simulink model "plant"  (R2023a)
settings: Solver=FixedStepAuto  StartTime=0.0  StopTime=10.0  FixedStep=0.01  RelTol=1e-3
libraries: shared6dof x1, simulink x1
settings Model: Creator=timme  LastModifiedBy=timme
settings OptimizationCC: BlockReduction=off  DefaultParameterBehavior=Inlined  BufferReuse=off

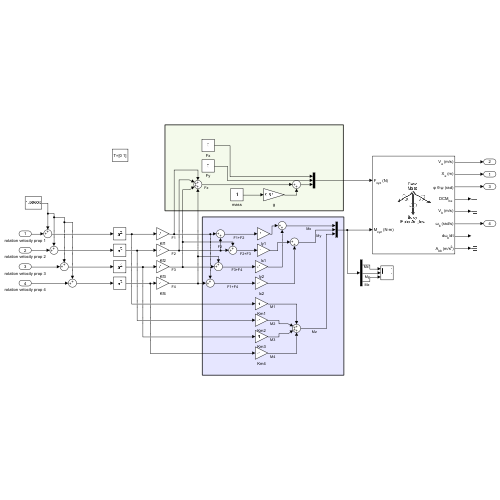
[thumbnail: Simulink's stored preview of the top-level diagram]
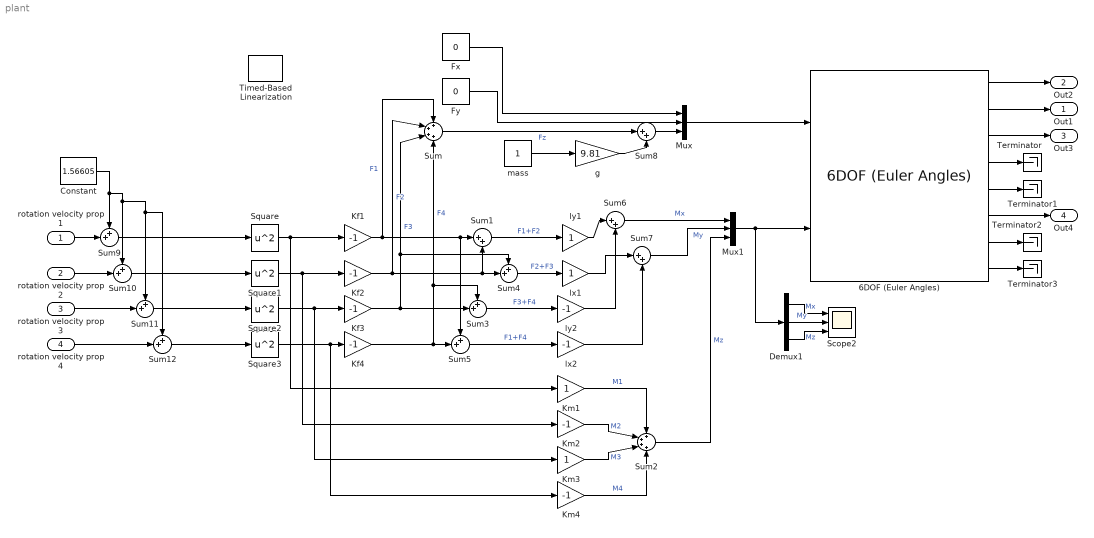
== system plant ==
  rotation velocity prop 1 : Inport
  rotation velocity prop 2 : Inport  Port=2
  rotation velocity prop 3 : Inport  Port=3
  rotation velocity prop 4 : Inport  Port=4
  6DOF (Euler Angles) : shared6dof/6DOF (Euler Angles)  units=Metric (MKS)  mtype=Fixed  rep=Euler Angles  xme_0=[0 0 0]  Vm_0=[0 0 0]  eul_0=[0 0 0]  pm_0=[0 0 0]  mass_0=1.0  mass_e=0.5  mass_f=2.0  inertia=eye(3)  inertia_e=eye(3)  inertia_f=2*eye(3)  k_quat=1.0  vre_flag=on  abi_flag=off  aMode=0  xme_statename=''  Vm_statename=''  eul_statename=''  quat_statename=''  pm_statename=''  mass_statename=''
  Constant : Constant  Value=1.56605
  Demux1 : Demux  Outputs=3
  Fx : Constant  Value=0
  Fy : Constant  Value=0
  Kf{1..4} (4 alike) : Gain  Gain=-1
  Km1 : Gain
  Km2 : Gain  Gain=-1
  Km3 : Gain
  Km4 : Gain  Gain=-1
  Mux : Mux  Inputs=3
  Mux1 : Mux  Inputs=3
  Scope2 : Scope  NumInputPorts=3
  Square{,1..3} (4 alike) : Math  Operator=square
  Sum : Sum  Inputs=++++
  Sum{1,6..8} (4 alike) : Sum  Inputs=|++
  Sum{3..5,9..12} (7 alike) : Sum  Inputs=++|
  Sum2 : Sum  Inputs=++++
  Terminator{,1..3} (4 alike) : Terminator
  Timed-Based Linearization : simulink/Model-Wide Utilities/Timed-Based Linearization  LinearizationTime=[0 1]  SampleTime=0.01
  g : Gain  Gain=9.81
  lx1 : Gain
  lx2 : Gain  Gain=-1
  ly1 : Gain
  ly2 : Gain  Gain=-1
  mass : Constant
  Out1 : Outport
  Out2 : Outport  Port=2
  Out3 : Outport  Port=3
  Out4 : Outport  Port=4
  wires:
  6DOF (Euler Angles)/2 -> Out1/1
  6DOF (Euler Angles)/1 -> Out2/1
  Mux/1 -> 6DOF (Euler Angles)/1
  Square/1 -> Kf1/1, Km1/1
  Square1/1 -> Km2/1, Kf2/1
  Square2/1 -> Km3/1, Kf3/1
  Square3/1 -> Km4/1, Kf4/1
  Sum/1 -> Sum8/1  "Fz"
  Fx/1 -> Mux/1
  Fy/1 -> Mux/2
  Kf1/1 -> Sum/1, Sum1/1, Sum5/1  "F1"
  Kf2/1 -> Sum/2, Sum4/2, Sum1/2  "F2"
  Kf4/1 -> Sum/4, Sum3/1, Sum5/2  "F4"
  Kf3/1 -> Sum/3, Sum4/1, Sum3/2  "F3"
  Mux1/1 -> Demux1/1, 6DOF (Euler Angles)/2
  Km1/1 -> Sum2/1  "M1"
  Km2/1 -> Sum2/2  "M2"
  Km3/1 -> Sum2/3  "M3"
  Km4/1 -> Sum2/4  "M4"
  Sum2/1 -> Mux1/3  "Mz"
  Sum5/1 -> lx2/1  "F1+F4"
  Sum3/1 -> ly2/1  "F3+F4"
  Sum4/1 -> lx1/1  "F2+F3"
  Sum1/1 -> ly1/1  "F1+F2"
  ly1/1 -> Sum6/1
  ly2/1 -> Sum6/2
  Sum6/1 -> Mux1/1  "Mx"
  Sum7/1 -> Mux1/2  "My"
  lx1/1 -> Sum7/1
  lx2/1 -> Sum7/2
  6DOF (Euler Angles)/4 -> Terminator/1
  6DOF (Euler Angles)/5 -> Terminator1/1
  6DOF (Euler Angles)/7 -> Terminator2/1
  6DOF (Euler Angles)/8 -> Terminator3/1
  Demux1/2 -> Scope2/2  "My"
  Demux1/1 -> Scope2/1  "Mx"
  Demux1/3 -> Scope2/3  "Mz"
  Sum8/1 -> Mux/3
  mass/1 -> g/1
  g/1 -> Sum8/2
  rotation velocity prop 2/1 -> Sum10/2
  rotation velocity prop 3/1 -> Sum11/2
  6DOF (Euler Angles)/3 -> Out3/1
  rotation velocity prop 1/1 -> Sum9/2
  rotation velocity prop 4/1 -> Sum12/2
  6DOF (Euler Angles)/6 -> Out4/1
  Constant/1 -> Sum12/1, Sum11/1, Sum10/1, Sum9/1
  Sum9/1 -> Square/1
  Sum10/1 -> Square1/1
  Sum12/1 -> Square3/1
  Sum11/1 -> Square2/1
